simulink model "mrefrobotarm_modified_previous_y_previous_u_previous_ref_pert"  (R2018b)
settings: Solver=FixedStepAuto  StartTime=0.0  StopTime=10  RelTol=1e-3  AbsTol=1e-6
undefined symbols (not defined in the file or in its folder): cc, options
libraries: neural x714, simulink x1
(part 16 of 26)

== system mrefrobotarm_modified_previous_y_previous_u_previous_ref_pert/sd=0.001/Layer 3/Delays 1 ==
  "p{3}" : Inport  PortDimensions=30
      mask Display: e = 0.06;c1 = [120 230 180]/255;c2 = ([120 230 180]+0)/(256+128);c3 = ([120 230 180]+128)/(256+128);patch([0 1 1 0],[0 0 1 1],c1);patch([0 1 1 1-e 1-e 0+e],[0 0 1 1-e 0+e 0+e],c2);patch([0 0 1 1-e 0+e 0+e],[0 1 1 1-e 1-e 0+e],c3);plot([0 1 1 0 0],[0 0 1 1 0]);
  mux : Mux  Inputs=1
      mask Display: e = 0.06;c1 = [120 150 230]/255;c2 = ([120 150 230]+0)/383;c3 = ([120 150 230]+128)/383;patch([0 1 1 0],[0 0 1 1],c1);patch([0 1 1 1-e 1-e 0+e],[0 0 1 1-e 0+e 0+e],c2);patch([0 0 1 1-e 0+e 0+e],[0 1 1 1-e 1-e 0+e],c3);plot([0 1 1 0 0],[0 0 1 1 0]);disp('Mux')
  "pd{3,2}" : Outport
      mask Display: e = 0.06;c1 = [120 230 180]/255;c2 = ([120 230 180]+0)/(256+128);c3 = ([120 230 180]+128)/(256+128);patch([0 1 1 0],[0 0 1 1],c1);patch([0 1 1 1-e 1-e 0+e],[0 0 1 1-e 0+e 0+e],c2);patch([0 0 1 1-e 0+e 0+e],[0 1 1 1-e 1-e 0+e],c3);plot([0 1 1 0 0],[0 0 1 1 0]);
  wires:
  "p{3}"/1 -> mux/1
  mux/1 -> "pd{3,2}"/1

== system mrefrobotarm_modified_previous_y_previous_u_previous_ref_pert/sd=0.001/Layer 3/LW{3,2} ==
  "ad{3,2}" : Inport  PortDimensions=30
      mask Display: e = 0.06;c1 = [120 230 180]/255;c2 = ([120 230 180]+0)/(256+128);c3 = ([120 230 180]+128)/(256+128);patch([0 1 1 0],[0 0 1 1],c1);patch([0 1 1 1-e 1-e 0+e],[0 0 1 1-e 0+e 0+e],c2);patch([0 0 1 1-e 0+e 0+e],[0 1 1 1-e 1-e 0+e],c3);plot([0 1 1 0 0],[0 0 1 1 0]);
  "IW{3,2}(1,:)'" : Constant  Value=[0.304250419965523433152299048742861486971378326416015625;0.95608938967641721173862379146157763898372650146484375;-0.2250542230244740038447304186774999834597110748291015625;-0.376135044993470335494833989287144504487514495849609375;-0.360224620807265638600114243672578595578670501708984375;0.2485440476899242467911932408242137171328067779541015625;0.18074154334064018723182698522577993571758270263671875;0.61962682359605170123728612452396191656589508056640625;0.0357588659652837981273165723905549384653568267822265625;0.353427117509543753381962005732930265367031097412109375;-0.52284302582703034989464185855467803776264190673828125;0.50949095237763220023197163754957728087902069091796875;0.374040794085301941951371418326743878424167633056640625;0.197896815199246567384960826530004851520061492919921875;1.0512812586579978191281270483159460127353668212890625;-0.36376784116270599600539981111069209873676300048828125;-0.454120740612595719110089476089342497289180755615234375;0.12581443827087712694634547005989588797092437744140625;-0.376948829105310523335248262810637243092060089111328125;0.62281250099934537534096534727723337709903717041015625;0.05311656788595241207584507492356351576745510101318359375;0.1277557248193866012986319447009009309113025665283203125;0.55690370252313836640922772858175449073314666748046875;-0.31533285096310492701121575009892694652080535888671875;0.015452407351345322228386436336222686804831027984619140625;0.453882236656812654285175767654436640441417694091796875;0.1658841818010752533485430149085004813969135284423828125;0.66024990000905336984260429744608700275421142578125;-0.56965674732652937795052139335894025862216949462890625;0.90156546155150663057753490647883154451847076416015625]
      mask Display: e = 0.06;c1 = [120 150 230]/255;c2 = ([120 150 230]+0)/383;c3 = ([120 150 230]+128)/383;patch([0 1 1 0],[0 0 1 1],c1);patch([0 1 1 1-e 1-e 0+e],[0 0 1 1-e 0+e 0+e],c2);patch([0 0 1 1-e 0+e 0+e],[0 1 1 1-e 1-e 0+e],c3);plot([0 1 1 0 0],[0 0 1 1 0]);disp('weights');
  Mux : Mux  Inputs=1
      mask Display: e = 0.06;c1 = [120 150 230]/255;c2 = ([120 150 230]+0)/383;c3 = ([120 150 230]+128)/383;patch([0 1 1 0],[0 0 1 1],c1);patch([0 1 1 1-e 1-e 0+e],[0 0 1 1-e 0+e 0+e],c2);patch([0 0 1 1-e 0+e 0+e],[0 1 1 1-e 1-e 0+e],c3);plot([0 1 1 0 0],[0 0 1 1 0]);disp('Mux');
  dotprod1 : neural/Weight Functions/dotprod
  "lz{3,2}" : Outport
      mask Display: e = 0.06;c1 = [120 230 180]/255;c2 = ([120 230 180]+0)/(256+128);c3 = ([120 230 180]+128)/(256+128);patch([0 1 1 0],[0 0 1 1],c1);patch([0 1 1 1-e 1-e 0+e],[0 0 1 1-e 0+e 0+e],c2);patch([0 0 1 1-e 0+e 0+e],[0 1 1 1-e 1-e 0+e],c3);plot([0 1 1 0 0],[0 0 1 1 0]);
  wires:
  "IW{3,2}(1,:)'"/1 -> dotprod1/1
  "ad{3,2}"/1 -> dotprod1/2
  dotprod1/1 -> Mux/1
  Mux/1 -> "lz{3,2}"/1

== system mrefrobotarm_modified_previous_y_previous_u_previous_ref_pert/sd=0.01/Layer 1/Delays 1 ==
  "p{1}" : Inport  PortDimensions=10
      mask Display: e = 0.06;c1 = [120 230 180]/255;c2 = ([120 230 180]+0)/(256+128);c3 = ([120 230 180]+128)/(256+128);patch([0 1 1 0],[0 0 1 1],c1);patch([0 1 1 1-e 1-e 0+e],[0 0 1 1-e 0+e 0+e],c2);patch([0 0 1 1-e 0+e 0+e],[0 1 1 1-e 1-e 0+e],c3);plot([0 1 1 0 0],[0 0 1 1 0]);
  mux : Mux  Inputs=1
      mask Display: e = 0.06;c1 = [120 150 230]/255;c2 = ([120 150 230]+0)/383;c3 = ([120 150 230]+128)/383;patch([0 1 1 0],[0 0 1 1],c1);patch([0 1 1 1-e 1-e 0+e],[0 0 1 1-e 0+e 0+e],c2);patch([0 0 1 1-e 0+e 0+e],[0 1 1 1-e 1-e 0+e],c3);plot([0 1 1 0 0],[0 0 1 1 0]);disp('Mux')
  "pd{1,1}" : Outport
      mask Display: e = 0.06;c1 = [120 230 180]/255;c2 = ([120 230 180]+0)/(256+128);c3 = ([120 230 180]+128)/(256+128);patch([0 1 1 0],[0 0 1 1],c1);patch([0 1 1 1-e 1-e 0+e],[0 0 1 1-e 0+e 0+e],c2);patch([0 0 1 1-e 0+e 0+e],[0 1 1 1-e 1-e 0+e],c3);plot([0 1 1 0 0],[0 0 1 1 0]);
  wires:
  "p{1}"/1 -> mux/1
  mux/1 -> "pd{1,1}"/1

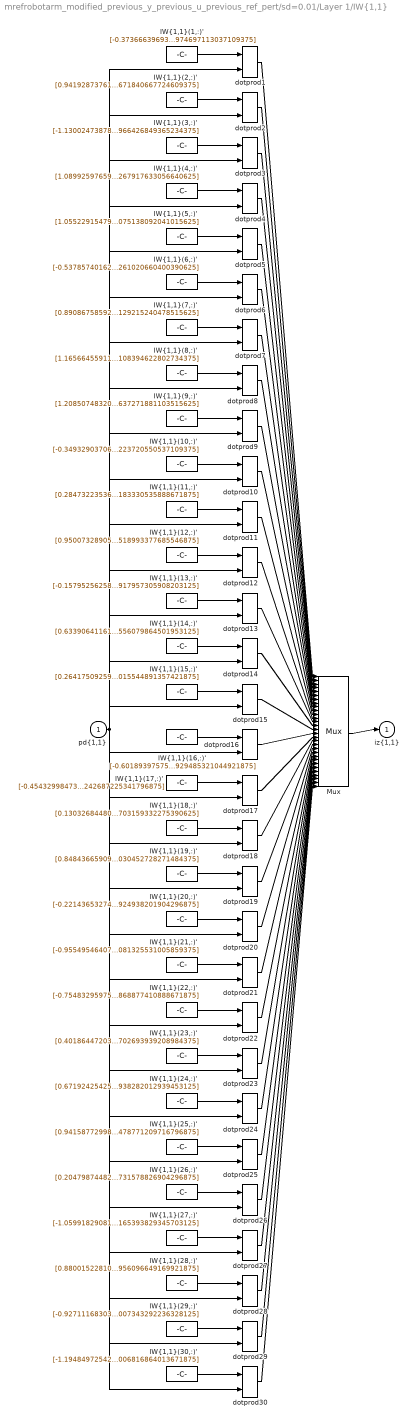
== system mrefrobotarm_modified_previous_y_previous_u_previous_ref_pert/sd=0.01/Layer 1/IW{1,1} ==
  "pd{1,1}" : Inport  PortDimensions=10
      mask Display: e = 0.06;c1 = [120 230 180]/255;c2 = ([120 230 180]+0)/(256+128);c3 = ([120 230 180]+128)/(256+128);patch([0 1 1 0],[0 0 1 1],c1);patch([0 1 1 1-e 1-e 0+e],[0 0 1 1-e 0+e 0+e],c2);patch([0 0 1 1-e 0+e 0+e],[0 1 1 1-e 1-e 0+e],c3);plot([0 1 1 0 0],[0 0 1 1 0]);
  "IW{1,1}(1,:)'" : Constant  Value=[-0.373666396932581801326733739188057370483875274658203125;0.8342126118727348771386687076301313936710357666015625;-0.011197072661472608212651635994916432537138462066650390625;-0.1189826779863965289241178879819926805794239044189453125;-0.43106244121923731338341667651548050343990325927734375;-0.65685372143279308065899613211513496935367584228515625;-0.70501077248312726819534645983367227017879486083984375;-0.66889030135945970467759025268605910241603851318359375;0.6178088380395170275960481376387178897857666015625;0.72227321164742619430398917756974697113037109375]
      mask Display: e = 0.06;c1 = [120 150 230]/255;c2 = ([120 150 230]+0)/383;c3 = ([120 150 230]+128)/383;patch([0 1 1 0],[0 0 1 1],c1);patch([0 1 1 1-e 1-e 0+e],[0 0 1 1-e 0+e 0+e],c2);patch([0 0 1 1-e 0+e 0+e],[0 1 1 1-e 1-e 0+e],c3);plot([0 1 1 0 0],[0 0 1 1 0]);disp('Weights');
  "IW{1,1}(10,:)'" : Constant  Value=[-0.34932903706578521951797711153631098568439483642578125;0.5754594486863415792043952023959718644618988037109375;0.17569160632102975849733184077194891870021820068359375;1.2952111243699615528157664812169969081878662109375;-0.436569519837344099943976516442489810287952423095703125;-1.394076235516755968291136014158837497234344482421875;0.435022388201156295917115812699194066226482391357421875;-0.35498042703611709658417794344131834805011749267578125;-0.6354671766612025596288049200666137039661407470703125;-0.41819219700407861406432630246854387223720550537109375]
      mask Display: e = 0.06;c1 = [120 150 230]/255;c2 = ([120 150 230]+0)/383;c3 = ([120 150 230]+128)/383;patch([0 1 1 0],[0 0 1 1],c1);patch([0 1 1 1-e 1-e 0+e],[0 0 1 1-e 0+e 0+e],c2);patch([0 0 1 1-e 0+e 0+e],[0 1 1 1-e 1-e 0+e],c3);plot([0 1 1 0 0],[0 0 1 1 0]);disp('Weights');
  "IW{1,1}(11,:)'" : Constant  Value=[0.284732235362669949818581471845391206443309783935546875;-1.09610049627214412026887657702900469303131103515625;0.73500064137660603424961891505517996847629547119140625;-0.88193299072955266826312481498462148010730743408203125;1.0396516913149149718975650102947838604450225830078125;-0.51605303056221207835818631792790256440639495849609375;0.394347831723694086658582591553567908704280853271484375;0.7559279312137838768848041581804864108562469482421875;0.1468331373809363682436668341324548237025737762451171875;0.65334699821204622605108625066350214183330535888671875]
      mask Display: e = 0.06;c1 = [120 150 230]/255;c2 = ([120 150 230]+0)/383;c3 = ([120 150 230]+128)/383;patch([0 1 1 0],[0 0 1 1],c1);patch([0 1 1 1-e 1-e 0+e],[0 0 1 1-e 0+e 0+e],c2);patch([0 0 1 1-e 0+e 0+e],[0 1 1 1-e 1-e 0+e],c3);plot([0 1 1 0 0],[0 0 1 1 0]);disp('Weights');
  "IW{1,1}(12,:)'" : Constant  Value=[0.95007328905688837039633654057979583740234375;0.6605105254338414777492971552419476211071014404296875;0.298050691228475328475866490407497622072696685791015625;-0.42415784928451716329078635681071318686008453369140625;-0.5535675844653307198228731067501939833164215087890625;0.050235947706228405162942607375953230075538158416748046875;0.174997796229193536277080056606791913509368896484375;-0.350519332110873105268211702423286624252796173095703125;0.351317294916767941526103413707460276782512664794921875;-0.24193035713773791695047066241386346518993377685546875]
      mask Display: e = 0.06;c1 = [120 150 230]/255;c2 = ([120 150 230]+0)/383;c3 = ([120 150 230]+128)/383;patch([0 1 1 0],[0 0 1 1],c1);patch([0 1 1 1-e 1-e 0+e],[0 0 1 1-e 0+e 0+e],c2);patch([0 0 1 1-e 0+e 0+e],[0 1 1 1-e 1-e 0+e],c3);plot([0 1 1 0 0],[0 0 1 1 0]);disp('Weights');
  "IW{1,1}(13,:)'" : Constant  Value=[-0.1579525625891935736166971082639065571129322052001953125;-0.288842840150287771816550730363815091550350189208984375;-1.2699052754012234434100037105963565409183502197265625;-0.0254421616350531086536701508293845108710229396820068359375;-0.12102797764330004703925425246779923327267169952392578125;0.7447562962196243585566435285727493464946746826171875;-1.2333942468134255765477291788556613028049468994140625;0.2266532156888579063735988938788068480789661407470703125;0.442939129814138576879400943653308786451816558837890625;0.002602153838740549514352284887763744336552917957305908203125]
      mask Display: e = 0.06;c1 = [120 150 230]/255;c2 = ([120 150 230]+0)/383;c3 = ([120 150 230]+128)/383;patch([0 1 1 0],[0 0 1 1],c1);patch([0 1 1 1-e 1-e 0+e],[0 0 1 1-e 0+e 0+e],c2);patch([0 0 1 1-e 0+e 0+e],[0 1 1 1-e 1-e 0+e],c3);plot([0 1 1 0 0],[0 0 1 1 0]);disp('Weights');
  "IW{1,1}(14,:)'" : Constant  Value=[0.63390641161183935992085025645792484283447265625;-0.06837840907831595205212948940243222750723361968994140625;0.31589468809984555530689931401866488158702850341796875;-0.81261587248496003343944948937860317528247833251953125;-1.045751467830205339026861111051402986049652099609375;0.047634147292226029779538265529481577686965465545654296875;1.0732644951763676832712235409417189657688140869140625;0.2263179537158319376555226654090802185237407684326171875;-1.009673481254381055549629309098236262798309326171875;-0.60537486558337694209086521368590183556079864501953125]
      mask Display: e = 0.06;c1 = [120 150 230]/255;c2 = ([120 150 230]+0)/383;c3 = ([120 150 230]+128)/383;patch([0 1 1 0],[0 0 1 1],c1);patch([0 1 1 1-e 1-e 0+e],[0 0 1 1-e 0+e 0+e],c2);patch([0 0 1 1-e 0+e 0+e],[0 1 1 1-e 1-e 0+e],c3);plot([0 1 1 0 0],[0 0 1 1 0]);disp('Weights');
  "IW{1,1}(15,:)'" : Constant  Value=[0.26417509259049054559653768592397682368755340576171875;0.83898437613462573114730957968276925384998321533203125;0.652733071824829647056276371586136519908905029296875;-1.2303025930992641523431530004017986357212066650390625;-0.647687402955962721051719199749641120433807373046875;-0.554948065545312285706813781871460378170013427734375;0.12005880031404271568451491702944622375071048736572265625;1.4364607707963277238860655415919609367847442626953125;-0.282416937459900818652158704935573041439056396484375;-1.580563027332878345276867548818700015544891357421875]
      mask Display: e = 0.06;c1 = [120 150 230]/255;c2 = ([120 150 230]+0)/383;c3 = ([120 150 230]+128)/383;patch([0 1 1 0],[0 0 1 1],c1);patch([0 1 1 1-e 1-e 0+e],[0 0 1 1-e 0+e 0+e],c2);patch([0 0 1 1-e 0+e 0+e],[0 1 1 1-e 1-e 0+e],c3);plot([0 1 1 0 0],[0 0 1 1 0]);disp('Weights');
  "IW{1,1}(16,:)'" : Constant  Value=[-0.60189397575390557459940055196057073771953582763671875;-0.0633492374733248542195696018097805790603160858154296875;0.3344783471988439504940515689668245613574981689453125;0.6228169089149926396231649050605483353137969970703125;0.428458195892239268598444823510362766683101654052734375;-0.1190580379975643421364139840079587884247303009033203125;-0.407579865337856561691154411164461635053157806396484375;1.8579085001480322159039815232972614467144012451171875;0.77822508833561609975504325120709836483001708984375;-0.6906604004046250633308545729960314929485321044921875]
      mask Display: e = 0.06;c1 = [120 150 230]/255;c2 = ([120 150 230]+0)/383;c3 = ([120 150 230]+128)/383;patch([0 1 1 0],[0 0 1 1],c1);patch([0 1 1 1-e 1-e 0+e],[0 0 1 1-e 0+e 0+e],c2);patch([0 0 1 1-e 0+e 0+e],[0 1 1 1-e 1-e 0+e],c3);plot([0 1 1 0 0],[0 0 1 1 0]);disp('Weights');
  "IW{1,1}(17,:)'" : Constant  Value=[-0.454329984731462743763330536239664070308208465576171875;-0.570146777419879402515334732015617191791534423828125;0.039859211471244819502413037071164580993354320526123046875;0.75297744596905047398394117408315651118755340576171875;0.127590539601346308895557513096719048917293548583984375;1.379878841001054734505260057630948722362518310546875;1.005532611684252675132711374317295849323272705078125;0.38024480425734186184172358480282127857208251953125;-0.84675268988207441633875305342371575534343719482421875;-0.287040336251347116824916838595527224242687225341796875]
      mask Display: e = 0.06;c1 = [120 150 230]/255;c2 = ([120 150 230]+0)/383;c3 = ([120 150 230]+128)/383;patch([0 1 1 0],[0 0 1 1],c1);patch([0 1 1 1-e 1-e 0+e],[0 0 1 1-e 0+e 0+e],c2);patch([0 0 1 1-e 0+e 0+e],[0 1 1 1-e 1-e 0+e],c3);plot([0 1 1 0 0],[0 0 1 1 0]);disp('Weights');
  "IW{1,1}(18,:)'" : Constant  Value=[0.1303268448018168601532096317896503023803234100341796875;-0.1764539738592298678820924351384746842086315155029296875;-0.1830953726063713482563599654895369894802570343017578125;-0.62533357703662140192335527899558655917644500732421875;0.283060963237438067974238720125867985188961029052734375;1.1659578304274209603619283370790071785449981689453125;-0.4972131470175151779500311022275127470493316650390625;-0.435982645988416572802037762812688015401363372802734375;-1.02275606117698014685402085888199508190155029296875;0.097981616678674721132580316407256759703159332275390625]
      mask Display: e = 0.06;c1 = [120 150 230]/255;c2 = ([120 150 230]+0)/383;c3 = ([120 150 230]+128)/383;patch([0 1 1 0],[0 0 1 1],c1);patch([0 1 1 1-e 1-e 0+e],[0 0 1 1-e 0+e 0+e],c2);patch([0 0 1 1-e 0+e 0+e],[0 1 1 1-e 1-e 0+e],c3);plot([0 1 1 0 0],[0 0 1 1 0]);disp('Weights');
  "IW{1,1}(19,:)'" : Constant  Value=[0.8484366590998266843826058902777731418609619140625;-0.089555197560177102200640320006641559302806854248046875;-0.96083919659357663878296307302662171423435211181640625;-0.324048843310693779340425635382416658103466033935546875;0.751873062542838255239985301159322261810302734375;0.5161090187603154522122395064798183739185333251953125;0.03291611590362542028032066809828393161296844482421875;0.04683261594865235910578604716647532768547534942626953125;-0.56719041806716818943101543482043780386447906494140625;0.518200102747657265211955746053718030452728271484375]
      mask Display: e = 0.06;c1 = [120 150 230]/255;c2 = ([120 150 230]+0)/383;c3 = ([120 150 230]+128)/383;patch([0 1 1 0],[0 0 1 1],c1);patch([0 1 1 1-e 1-e 0+e],[0 0 1 1-e 0+e 0+e],c2);patch([0 0 1 1-e 0+e 0+e],[0 1 1 1-e 1-e 0+e],c3);plot([0 1 1 0 0],[0 0 1 1 0]);disp('Weights');
  "IW{1,1}(2,:)'" : Constant  Value=[0.941928737611533950513376112212426960468292236328125;0.68716008339049661213238096024724654853343963623046875;-0.55613620646828654248139400806394405663013458251953125;-0.68892585732646083318542196138878352940082550048828125;-0.03233186205985331962420303852923098020255565643310546875;0.86536151012683848460227409304934553802013397216796875;1.0499230895233313543002395817893557250499725341796875;0.656453850983135023255954365595243871212005615234375;0.48135080235902538703385289409197866916656494140625;-0.271833773490931240868206941740936599671840667724609375]
      mask Display: e = 0.06;c1 = [120 150 230]/255;c2 = ([120 150 230]+0)/383;c3 = ([120 150 230]+128)/383;patch([0 1 1 0],[0 0 1 1],c1);patch([0 1 1 1-e 1-e 0+e],[0 0 1 1-e 0+e 0+e],c2);patch([0 0 1 1-e 0+e 0+e],[0 1 1 1-e 1-e 0+e],c3);plot([0 1 1 0 0],[0 0 1 1 0]);disp('Weights');
  "IW{1,1}(20,:)'" : Constant  Value=[-0.2214365327418121032199138653595582582056522369384765625;-0.1825122835922346198334054179213126190006732940673828125;0.94269643651769197134626665501855313777923583984375;0.66989709606531333552226215033442713320255279541015625;-0.91110487383422888996165056596510112285614013671875;0.0766897662633689025657446336481370963156223297119140625;0.316023435171211397598511894102557562291622161865234375;-0.128000498766459747113088951664394699037075042724609375;0.70567274052382311655406965655856765806674957275390625;0.85332160184190175566953939778613857924938201904296875]
      mask Display: e = 0.06;c1 = [120 150 230]/255;c2 = ([120 150 230]+0)/383;c3 = ([120 150 230]+128)/383;patch([0 1 1 0],[0 0 1 1],c1);patch([0 1 1 1-e 1-e 0+e],[0 0 1 1-e 0+e 0+e],c2);patch([0 0 1 1-e 0+e 0+e],[0 1 1 1-e 1-e 0+e],c3);plot([0 1 1 0 0],[0 0 1 1 0]);disp('Weights');
  "IW{1,1}(21,:)'" : Constant  Value=[-0.95549546407072327713905224300106056034564971923828125;0.1179762331301006106354378744072164408862590789794921875;-0.09861128785628960058406988764545531012117862701416015625;-0.54057080772691257219975113912369124591350555419921875;-0.66947841207596237023125240739318542182445526123046875;-0.32618027842415353578786607613437809050083160400390625;0.74605385520855216352487104813917540013790130615234375;-0.25728988916763106953311535107786767184734344482421875;-0.43768192014666651434851019075722433626651763916015625;0.728564116249044158024616990587674081325531005859375]
      mask Display: e = 0.06;c1 = [120 150 230]/255;c2 = ([120 150 230]+0)/383;c3 = ([120 150 230]+128)/383;patch([0 1 1 0],[0 0 1 1],c1);patch([0 1 1 1-e 1-e 0+e],[0 0 1 1-e 0+e 0+e],c2);patch([0 0 1 1-e 0+e 0+e],[0 1 1 1-e 1-e 0+e],c3);plot([0 1 1 0 0],[0 0 1 1 0]);disp('Weights');
  "IW{1,1}(22,:)'" : Constant  Value=[-0.7548329597524683354237140520126558840274810791015625;-0.7319418005360487367028099470189772546291351318359375;-0.290849879008257372614565383628359995782375335693359375;-0.463380838296664487874210180962109006941318511962890625;1.1255998063561367672491542180068790912628173828125;-0.97038555432252671106851948934490792453289031982421875;-0.164098414965231587103744459454901516437530517578125;-0.62132749819644816913211116116144694387912750244140625;-0.1927284153706785574389215298651834018528461456298828125;0.488807831002793846675302802395890466868877410888671875]
      mask Display: e = 0.06;c1 = [120 150 230]/255;c2 = ([120 150 230]+0)/383;c3 = ([120 150 230]+128)/383;patch([0 1 1 0],[0 0 1 1],c1);patch([0 1 1 1-e 1-e 0+e],[0 0 1 1-e 0+e 0+e],c2);patch([0 0 1 1-e 0+e 0+e],[0 1 1 1-e 1-e 0+e],c3);plot([0 1 1 0 0],[0 0 1 1 0]);disp('Weights');
  "IW{1,1}(23,:)'" : Constant  Value=[0.401864472030851904715831324210739694535732269287109375;-0.0086770385377600255105701165803111507557332515716552734375;0.60710704444556196079929577535949647426605224609375;-0.5376108123680392036902730978908948600292205810546875;-0.10059065297415172024475538137266994453966617584228515625;1.199528892981079675195132949738763272762298583984375;-1.0236977579446691066777930245734751224517822265625;-0.06335088635064857476297817129307077266275882720947265625;-0.546474215400909457684974768199026584625244140625;-0.78345537643438889485736353890388272702693939208984375]
      mask Display: e = 0.06;c1 = [120 150 230]/255;c2 = ([120 150 230]+0)/383;c3 = ([120 150 230]+128)/383;patch([0 1 1 0],[0 0 1 1],c1);patch([0 1 1 1-e 1-e 0+e],[0 0 1 1-e 0+e 0+e],c2);patch([0 0 1 1-e 0+e 0+e],[0 1 1 1-e 1-e 0+e],c3);plot([0 1 1 0 0],[0 0 1 1 0]);disp('Weights');
  "IW{1,1}(24,:)'" : Constant  Value=[0.67192425425232171765088651227415539324283599853515625;-0.117973980594329341808901290278299711644649505615234375;-0.42144959176436069814286611290299333631992340087890625;1.1287148061228802209399191269767470657825469970703125;0.336085001581777176316023769686580635607242584228515625;-0.55173387916368599181993204183527268469333648681640625;0.1443114999876366211228884139927686192095279693603515625;-1.11205329635469229998534501646645367145538330078125;0.8616911363802632894959288023528642952442169189453125;-0.361000947585930209715598948605475015938282012939453125]
      mask Display: e = 0.06;c1 = [120 150 230]/255;c2 = ([120 150 230]+0)/383;c3 = ([120 150 230]+128)/383;patch([0 1 1 0],[0 0 1 1],c1);patch([0 1 1 1-e 1-e 0+e],[0 0 1 1-e 0+e 0+e],c2);patch([0 0 1 1-e 0+e 0+e],[0 1 1 1-e 1-e 0+e],c3);plot([0 1 1 0 0],[0 0 1 1 0]);disp('Weights');
  "IW{1,1}(25,:)'" : Constant  Value=[0.94158772998720452473975228713243268430233001708984375;-0.355300580924523934367442734583164565265178680419921875;-0.9066246013285661486946764853200875222682952880859375;-0.2475892563421986658500628664114628918468952178955078125;-0.8075537348354961952878738884464837610721588134765625;0.25452072216826271411349580375826917588710784912109375;1.1492322317977119450205236717010848224163055419921875;-0.66339890208506357982543022444588132202625274658203125;-0.189957307261183760971334777423180639743804931640625;0.69062211649628846288351269322447478771209716796875]
      mask Display: e = 0.06;c1 = [120 150 230]/255;c2 = ([120 150 230]+0)/383;c3 = ([120 150 230]+128)/383;patch([0 1 1 0],[0 0 1 1],c1);patch([0 1 1 1-e 1-e 0+e],[0 0 1 1-e 0+e 0+e],c2);patch([0 0 1 1-e 0+e 0+e],[0 1 1 1-e 1-e 0+e],c3);plot([0 1 1 0 0],[0 0 1 1 0]);disp('Weights');
  "IW{1,1}(26,:)'" : Constant  Value=[0.204798744827981715754816605112864635884761810302734375;1.071172011255632217086031232611276209354400634765625;-0.9348182552544590517840106258518062531948089599609375;-0.47504187577336998149490909781889058649539947509765625;-0.1861969629034221640484503268453408963978290557861328125;-0.8825310306384734904128208654583431780338287353515625;0.2308417658754307877355671507757506333291530609130859375;-1.031252749757456843582303918083198368549346923828125;-0.95110708096078011575258415177813731133937835693359375;0.048197947580719817384231618007106590084731578826904296875]
      mask Display: e = 0.06;c1 = [120 150 230]/255;c2 = ([120 150 230]+0)/383;c3 = ([120 150 230]+128)/383;patch([0 1 1 0],[0 0 1 1],c1);patch([0 1 1 1-e 1-e 0+e],[0 0 1 1-e 0+e 0+e],c2);patch([0 0 1 1-e 0+e 0+e],[0 1 1 1-e 1-e 0+e],c3);plot([0 1 1 0 0],[0 0 1 1 0]);disp('Weights');
  "IW{1,1}(27,:)'" : Constant  Value=[-1.0599182908146740356158943541231565177440643310546875;1.1109888126790481432948354267864488065242767333984375;0.5610324564643220934812006817082874476909637451171875;-0.71467691183178982949897317666909657418727874755859375;0.3426830929529651736942241768701933324337005615234375;0.98446403161817264138022665065363980829715728759765625;0.89315444135654764590270815460826270282268524169921875;0.397595320232244808789090484424377791583538055419921875;0.99104080535155125719626312275067903101444244384765625;-0.5277859566275762137621541114640422165393829345703125]
      mask Display: e = 0.06;c1 = [120 150 230]/255;c2 = ([120 150 230]+0)/383;c3 = ([120 150 230]+128)/383;patch([0 1 1 0],[0 0 1 1],c1);patch([0 1 1 1-e 1-e 0+e],[0 0 1 1-e 0+e 0+e],c2);patch([0 0 1 1-e 0+e 0+e],[0 1 1 1-e 1-e 0+e],c3);plot([0 1 1 0 0],[0 0 1 1 0]);disp('Weights');
  "IW{1,1}(28,:)'" : Constant  Value=[0.88001522810452492695532100697164423763751983642578125;-0.69354451180706877533310716898995451629161834716796875;-0.811402949666907513659452888532541692256927490234375;0.71703026438105255113697467095335014164447784423828125;-0.47863890374426010243524842735496349632740020751953125;-0.98011176245736308931810754074831493198871612548828125;0.77736246409221421149737807354540564119815826416015625;-0.814279752905500142645678351982496678829193115234375;-0.5813106650136570241471645204001106321811676025390625;-0.48435319686551714379874056248809210956096649169921875]
      mask Display: e = 0.06;c1 = [120 150 230]/255;c2 = ([120 150 230]+0)/383;c3 = ([120 150 230]+128)/383;patch([0 1 1 0],[0 0 1 1],c1);patch([0 1 1 1-e 1-e 0+e],[0 0 1 1-e 0+e 0+e],c2);patch([0 0 1 1-e 0+e 0+e],[0 1 1 1-e 1-e 0+e],c3);plot([0 1 1 0 0],[0 0 1 1 0]);disp('Weights');
  "IW{1,1}(29,:)'" : Constant  Value=[-0.92711168303679525326543853225302882492542266845703125;0.19849326015858970162497598721529357135295867919921875;-0.72142842897595993445492013051989488303661346435546875;0.23047616633720746648350541363470256328582763671875;-1.0850921510199171837740550472517497837543487548828125;-0.58492654767090501710669059320935048162937164306640625;-0.6851769451629448060003824139130301773548126220703125;1.47439836974424931526073123677633702754974365234375;1.0267940316156722868612405363819561898708343505859375;-0.60267815461566431878281946410425007343292236328125]
      mask Display: e = 0.06;c1 = [120 150 230]/255;c2 = ([120 150 230]+0)/383;c3 = ([120 150 230]+128)/383;patch([0 1 1 0],[0 0 1 1],c1);patch([0 1 1 1-e 1-e 0+e],[0 0 1 1-e 0+e 0+e],c2);patch([0 0 1 1-e 0+e 0+e],[0 1 1 1-e 1-e 0+e],c3);plot([0 1 1 0 0],[0 0 1 1 0]);disp('Weights');
  "IW{1,1}(3,:)'" : Constant  Value=[-1.130024738780765591883437082287855446338653564453125;-0.043119209665583128898713738408332574181258678436279296875;-0.67010275490164161737993708811700344085693359375;0.433711657622901480824140207914751954376697540283203125;1.244678469438450729711576059344224631786346435546875;0.410817839651130167766268641571514308452606201171875;0.196431034858671527132401024573482573032379150390625;-0.00710842355936054486054143097817359375767409801483154296875;0.870799870747253290659273261553607881069183349609375;1.4490229887895773597250581588014028966426849365234375]
      mask Display: e = 0.06;c1 = [120 150 230]/255;c2 = ([120 150 230]+0)/383;c3 = ([120 150 230]+128)/383;patch([0 1 1 0],[0 0 1 1],c1);patch([0 1 1 1-e 1-e 0+e],[0 0 1 1-e 0+e 0+e],c2);patch([0 0 1 1-e 0+e 0+e],[0 1 1 1-e 1-e 0+e],c3);plot([0 1 1 0 0],[0 0 1 1 0]);disp('Weights');
  "IW{1,1}(30,:)'" : Constant  Value=[-1.1948497254284176083416468827635981142520904541015625;-0.8910875231320745104568459282745607197284698486328125;0.551999046957500905108418010058812797069549560546875;-0.07579123075997451497443080370430834591388702392578125;-0.92273617727313317349313592785620130598545074462890625;-0.20942889920231977374243115264107473194599151611328125;0.65640814824983639841349258858826942741870880126953125;0.00805092094773116918882127635015422129072248935699462890625;0.68163122232695971813853930143523029983043670654296875;0.09605977590857998904549930330176721327006816864013671875]
      mask Display: e = 0.06;c1 = [120 150 230]/255;c2 = ([120 150 230]+0)/383;c3 = ([120 150 230]+128)/383;patch([0 1 1 0],[0 0 1 1],c1);patch([0 1 1 1-e 1-e 0+e],[0 0 1 1-e 0+e 0+e],c2);patch([0 0 1 1-e 0+e 0+e],[0 1 1 1-e 1-e 0+e],c3);plot([0 1 1 0 0],[0 0 1 1 0]);disp('Weights');
  "IW{1,1}(4,:)'" : Constant  Value=[1.08992597659519407926609346759505569934844970703125;-0.58237987125583623448932257815613411366939544677734375;-0.363021619608467627227099683295818977057933807373046875;-0.339292594654479306992556075783795677125453948974609375;0.61918413796120475023343487919191829860210418701171875;-0.9725681955654430499436102763866074383258819580078125;1.1039034325732723917923294720822013914585113525390625;0.0741447906027425662767171843370306305587291717529296875;0.0675753702505202669126305181634961627423763275146484375;-0.73681662575161654959998713820823468267917633056640625]
      mask Display: e = 0.06;c1 = [120 150 230]/255;c2 = ([120 150 230]+0)/383;c3 = ([120 150 230]+128)/383;patch([0 1 1 0],[0 0 1 1],c1);patch([0 1 1 1-e 1-e 0+e],[0 0 1 1-e 0+e 0+e],c2);patch([0 0 1 1-e 0+e 0+e],[0 1 1 1-e 1-e 0+e],c3);plot([0 1 1 0 0],[0 0 1 1 0]);disp('Weights');
  "IW{1,1}(5,:)'" : Constant  Value=[1.0552291547940868543520309685845859348773956298828125;-1.104812136932537658395858670701272785663604736328125;0.72873393389660090502246703181299380958080291748046875;-0.8612030454344881125194888227269984781742095947265625;-0.3027063153814761875537442392669618129730224609375;-0.07698512289075974679430913738542585633695125579833984375;-0.417815446570052706487530258527840487658977508544921875;-0.178589070035018393500791944461525417864322662353515625;-0.76757793018494668846329886946477927267551422119140625;0.1262519523740535110079008518368937075138092041015625]
      mask Display: e = 0.06;c1 = [120 150 230]/255;c2 = ([120 150 230]+0)/383;c3 = ([120 150 230]+128)/383;patch([0 1 1 0],[0 0 1 1],c1);patch([0 1 1 1-e 1-e 0+e],[0 0 1 1-e 0+e 0+e],c2);patch([0 0 1 1-e 0+e 0+e],[0 1 1 1-e 1-e 0+e],c3);plot([0 1 1 0 0],[0 0 1 1 0]);disp('Weights');
  "IW{1,1}(6,:)'" : Constant  Value=[-0.53785740162570350175741396014927886426448822021484375;1.0202764905407075701759822550229728221893310546875;0.75740734171249168849016086824121885001659393310546875;0.6364853769874592170907590116257779300212860107421875;0.78675801278199475330410450624185614287853240966796875;-2.025018975438089174900824218639172613620758056640625;-0.04466141888967088691142492962171672843396663665771484375;-1.12396153465951531558175702230073511600494384765625;1.700423243584629151570197791443206369876861572265625;0.054192449983166836313674963321318500675261020660400390625]
      mask Display: e = 0.06;c1 = [120 150 230]/255;c2 = ([120 150 230]+0)/383;c3 = ([120 150 230]+128)/383;patch([0 1 1 0],[0 0 1 1],c1);patch([0 1 1 1-e 1-e 0+e],[0 0 1 1-e 0+e 0+e],c2);patch([0 0 1 1-e 0+e 0+e],[0 1 1 1-e 1-e 0+e],c3);plot([0 1 1 0 0],[0 0 1 1 0]);disp('Weights');
  "IW{1,1}(7,:)'" : Constant  Value=[0.8908675859259449492100202405708841979503631591796875;-0.32538955288765902817971209515235386788845062255859375;-0.8641033883707140983432282155263237655162811279296875;-0.63417231703426579780824567933450452983379364013671875;-1.0923460059077718664610756604815833270549774169921875;0.79585959966494235207079555038944818079471588134765625;0.804653844402537288260646164417266845703125;1.6006171295811275623321989769465290009975433349609375;0.5229533898641733902223904806305654346942901611328125;-0.82014240507356517273507279242039658129215240478515625]
      mask Display: e = 0.06;c1 = [120 150 230]/255;c2 = ([120 150 230]+0)/383;c3 = ([120 150 230]+128)/383;patch([0 1 1 0],[0 0 1 1],c1);patch([0 1 1 1-e 1-e 0+e],[0 0 1 1-e 0+e 0+e],c2);patch([0 0 1 1-e 0+e 0+e],[0 1 1 1-e 1-e 0+e],c3);plot([0 1 1 0 0],[0 0 1 1 0]);disp('Weights');
  "IW{1,1}(8,:)'" : Constant  Value=[1.1656645591101864045668889957596547901630401611328125;-0.318177656617735060695650872730766423046588897705078125;-0.4659149656588781329702442235429771244525909423828125;-0.25512673934292962041325836253236047923564910888671875;-0.6137093296096465255828888984979130327701568603515625;0.5604147283024125680839233609731309115886688232421875;-0.89921120975476320769104177088593132793903350830078125;0.8895682605237895668182090957998298108577728271484375;0.27615501683535448318451699378783814609050750732421875;0.4989566887383227733465673736645840108394622802734375]
      mask Display: e = 0.06;c1 = [120 150 230]/255;c2 = ([120 150 230]+0)/383;c3 = ([120 150 230]+128)/383;patch([0 1 1 0],[0 0 1 1],c1);patch([0 1 1 1-e 1-e 0+e],[0 0 1 1-e 0+e 0+e],c2);patch([0 0 1 1-e 0+e 0+e],[0 1 1 1-e 1-e 0+e],c3);plot([0 1 1 0 0],[0 0 1 1 0]);disp('Weights');
  "IW{1,1}(9,:)'" : Constant  Value=[1.208507483207707178252121593686752021312713623046875;-0.28501973360403543011898364056833088397979736328125;0.975868366907793216569189098663628101348876953125;0.128148687595778465464491091552190482616424560546875;-0.34207568225799167560552405120688490569591522216796875;0.6780328830658268746134353932575322687625885009765625;0.1140906502179252768325312672459403984248638153076171875;-1.042840264426599272695739273331128060817718505859375;-0.60549546056487935086209972723736427724361419677734375;-0.8841670467524933574310352923930622637271881103515625]
      mask Display: e = 0.06;c1 = [120 150 230]/255;c2 = ([120 150 230]+0)/383;c3 = ([120 150 230]+128)/383;patch([0 1 1 0],[0 0 1 1],c1);patch([0 1 1 1-e 1-e 0+e],[0 0 1 1-e 0+e 0+e],c2);patch([0 0 1 1-e 0+e 0+e],[0 1 1 1-e 1-e 0+e],c3);plot([0 1 1 0 0],[0 0 1 1 0]);disp('Weights');
  Mux : Mux  Inputs=30
      mask Display: e = 0.06;c1 = [120 150 230]/255;c2 = ([120 150 230]+0)/383;c3 = ([120 150 230]+128)/383;patch([0 1 1 0],[0 0 1 1],c1);patch([0 1 1 1-e 1-e 0+e],[0 0 1 1-e 0+e 0+e],c2);patch([0 0 1 1-e 0+e 0+e],[0 1 1 1-e 1-e 0+e],c3);plot([0 1 1 0 0],[0 0 1 1 0]);disp('Mux');
  dotprod{1..30} (30 alike) : neural/Weight Functions/dotprod
  "iz{1,1}" : Outport
      mask Display: e = 0.06;c1 = [120 230 180]/255;c2 = ([120 230 180]+0)/(256+128);c3 = ([120 230 180]+128)/(256+128);patch([0 1 1 0],[0 0 1 1],c1);patch([0 1 1 1-e 1-e 0+e],[0 0 1 1-e 0+e 0+e],c2);patch([0 0 1 1-e 0+e 0+e],[0 1 1 1-e 1-e 0+e],c3);plot([0 1 1 0 0],[0 0 1 1 0]);
  wires:
  "IW{1,1}(1,:)'"/1 -> dotprod1/1
  "pd{1,1}"/1 -> dotprod1/2, dotprod2/2, dotprod3/2, dotprod4/2, dotprod5/2, dotprod6/2, dotprod7/2, dotprod8/2, dotprod9/2, dotprod10/2, dotprod11/2, dotprod12/2, dotprod13/2, dotprod14/2, dotprod15/2, dotprod16/2, dotprod17/2, dotprod18/2, dotprod19/2, dotprod20/2, dotprod21/2, dotprod22/2, dotprod23/2, dotprod24/2, dotprod25/2, dotprod26/2, dotprod27/2, dotprod28/2, dotprod29/2, dotprod30/2
  dotprod1/1 -> Mux/1
  "IW{1,1}(2,:)'"/1 -> dotprod2/1
  dotprod2/1 -> Mux/2
  "IW{1,1}(3,:)'"/1 -> dotprod3/1
  dotprod3/1 -> Mux/3
  "IW{1,1}(4,:)'"/1 -> dotprod4/1
  dotprod4/1 -> Mux/4
  "IW{1,1}(5,:)'"/1 -> dotprod5/1
  dotprod5/1 -> Mux/5
  "IW{1,1}(6,:)'"/1 -> dotprod6/1
  dotprod6/1 -> Mux/6
  "IW{1,1}(7,:)'"/1 -> dotprod7/1
  dotprod7/1 -> Mux/7
  "IW{1,1}(8,:)'"/1 -> dotprod8/1
  dotprod8/1 -> Mux/8
  "IW{1,1}(9,:)'"/1 -> dotprod9/1
  dotprod9/1 -> Mux/9
  "IW{1,1}(10,:)'"/1 -> dotprod10/1
  dotprod10/1 -> Mux/10
  "IW{1,1}(11,:)'"/1 -> dotprod11/1
  dotprod11/1 -> Mux/11
  "IW{1,1}(12,:)'"/1 -> dotprod12/1
  dotprod12/1 -> Mux/12
  "IW{1,1}(13,:)'"/1 -> dotprod13/1
  dotprod13/1 -> Mux/13
  "IW{1,1}(14,:)'"/1 -> dotprod14/1
  dotprod14/1 -> Mux/14
  "IW{1,1}(15,:)'"/1 -> dotprod15/1
  dotprod15/1 -> Mux/15
  "IW{1,1}(16,:)'"/1 -> dotprod16/1
  dotprod16/1 -> Mux/16
  "IW{1,1}(17,:)'"/1 -> dotprod17/1
  dotprod17/1 -> Mux/17
  "IW{1,1}(18,:)'"/1 -> dotprod18/1
  dotprod18/1 -> Mux/18
  "IW{1,1}(19,:)'"/1 -> dotprod19/1
  dotprod19/1 -> Mux/19
  "IW{1,1}(20,:)'"/1 -> dotprod20/1
  dotprod20/1 -> Mux/20
  "IW{1,1}(21,:)'"/1 -> dotprod21/1
  dotprod21/1 -> Mux/21
  "IW{1,1}(22,:)'"/1 -> dotprod22/1
  dotprod22/1 -> Mux/22
  "IW{1,1}(23,:)'"/1 -> dotprod23/1
  dotprod23/1 -> Mux/23
  "IW{1,1}(24,:)'"/1 -> dotprod24/1
  dotprod24/1 -> Mux/24
  "IW{1,1}(25,:)'"/1 -> dotprod25/1
  dotprod25/1 -> Mux/25
  "IW{1,1}(26,:)'"/1 -> dotprod26/1
  dotprod26/1 -> Mux/26
  "IW{1,1}(27,:)'"/1 -> dotprod27/1
  dotprod27/1 -> Mux/27
  "IW{1,1}(28,:)'"/1 -> dotprod28/1
  dotprod28/1 -> Mux/28
  "IW{1,1}(29,:)'"/1 -> dotprod29/1
  dotprod29/1 -> Mux/29
  "IW{1,1}(30,:)'"/1 -> dotprod30/1
  dotprod30/1 -> Mux/30
  Mux/1 -> "iz{1,1}"/1

== system mrefrobotarm_modified_previous_y_previous_u_previous_ref_pert/sd=0.01/Layer 2/Delays 1 ==
  "p{2}" : Inport  PortDimensions=30
      mask Display: e = 0.06;c1 = [120 230 180]/255;c2 = ([120 230 180]+0)/(256+128);c3 = ([120 230 180]+128)/(256+128);patch([0 1 1 0],[0 0 1 1],c1);patch([0 1 1 1-e 1-e 0+e],[0 0 1 1-e 0+e 0+e],c2);patch([0 0 1 1-e 0+e 0+e],[0 1 1 1-e 1-e 0+e],c3);plot([0 1 1 0 0],[0 0 1 1 0]);
  mux : Mux  Inputs=1
      mask Display: e = 0.06;c1 = [120 150 230]/255;c2 = ([120 150 230]+0)/383;c3 = ([120 150 230]+128)/383;patch([0 1 1 0],[0 0 1 1],c1);patch([0 1 1 1-e 1-e 0+e],[0 0 1 1-e 0+e 0+e],c2);patch([0 0 1 1-e 0+e 0+e],[0 1 1 1-e 1-e 0+e],c3);plot([0 1 1 0 0],[0 0 1 1 0]);disp('Mux')
  "pd{2,1}" : Outport
      mask Display: e = 0.06;c1 = [120 230 180]/255;c2 = ([120 230 180]+0)/(256+128);c3 = ([120 230 180]+128)/(256+128);patch([0 1 1 0],[0 0 1 1],c1);patch([0 1 1 1-e 1-e 0+e],[0 0 1 1-e 0+e 0+e],c2);patch([0 0 1 1-e 0+e 0+e],[0 1 1 1-e 1-e 0+e],c3);plot([0 1 1 0 0],[0 0 1 1 0]);
  wires:
  "p{2}"/1 -> mux/1
  mux/1 -> "pd{2,1}"/1
